simulink subsystem "Controller"  (R2022b)
settings: Solver=VariableStepAuto  StartTime=0.0  StopTime=10.0  RelTol=1e-3
libraries: arduinomotorcarrierlib x1
settings Model: Creator=domin  LastModifiedBy=domin

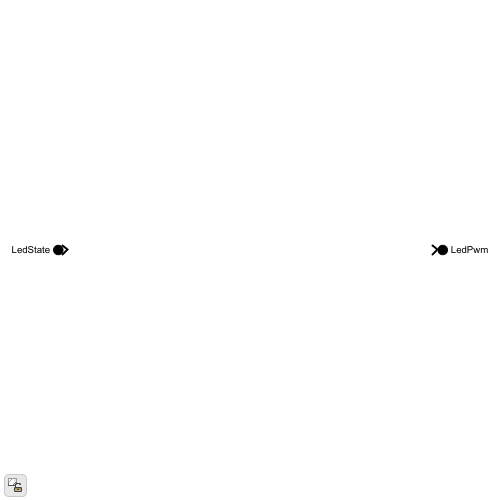
[thumbnail: Simulink's stored preview of the top-level diagram]
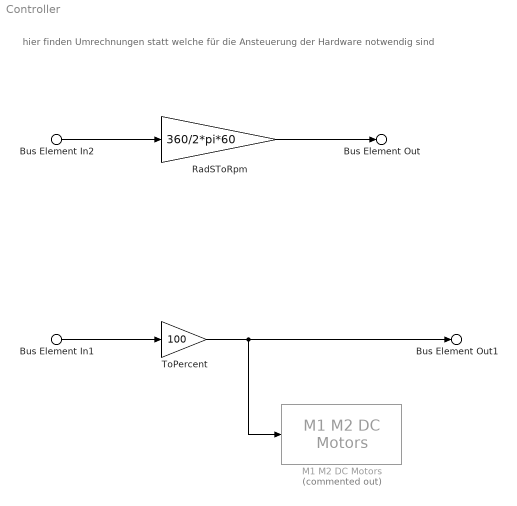
== system Controller ==
  note: hier finden Umrechnungen statt welche für die Ansteuerung der Hardware notwendig sind
  Bus Element In2 : Inport  PortName=MotorRadS
  Bus Element In1 : Inport  Port=2  PortName=MotorSetpoint
  M1 M2 DC Motors : arduinomotorcarrierlib/M1 M2 DC Motors  Commented=on  SlaveAddress=uint8( hex2dec( '66' ) )  blockPlatform=ARDUINO  MotorNumber=M1  MotorCarrierPWMFreq=100
  RadSToRpm : Gain  Gain=360/2*pi*60
  ToPercent : Gain  Gain=100
  Bus Element Out1 : Outport  PortName=MotorSetpointPercent
  Bus Element Out : Outport  Port=2  PortName=MotorRpm
  wires:
  Bus Element In1/1 -> ToPercent/1
  ToPercent/1 -> Bus Element Out1/1, M1 M2 DC Motors/1
  Bus Element In2/1 -> RadSToRpm/1
  RadSToRpm/1 -> Bus Element Out/1
